simulink model "Multiple"  (R2023a)
settings: Solver=VariableStepAuto  StartTime=0.0  StopTime=1  RelTol=1e-3
settings Model: Creator=Admin  LastModifiedBy=Admin

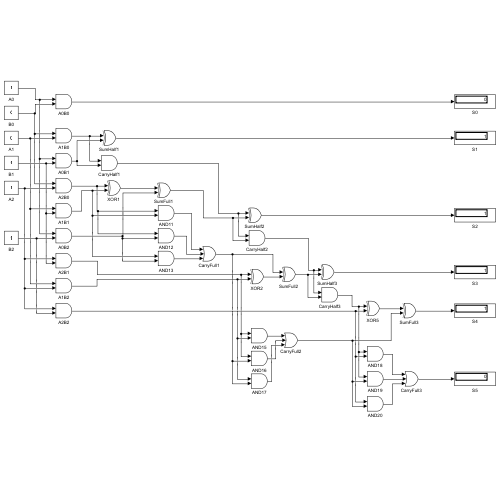
[thumbnail: Simulink's stored preview of the top-level diagram]
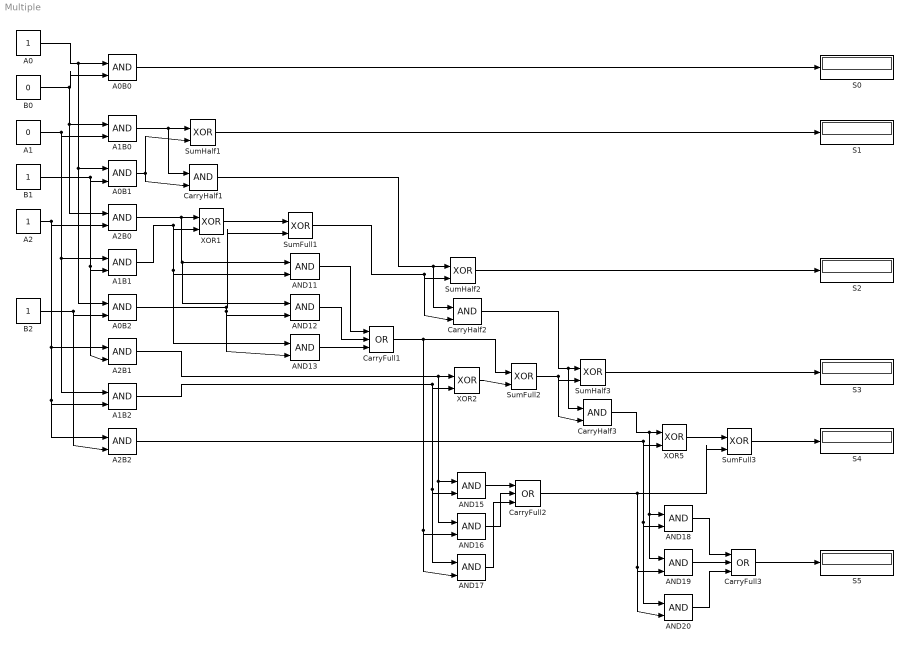
== system Multiple ==
  A0 : Constant  SampleTime=-1
  A0B0 : Logic  IconShape=distinctive  AllPortsSameDT=off  OutDataTypeStr=boolean
  A0B1 : Logic  IconShape=distinctive  AllPortsSameDT=off  OutDataTypeStr=boolean
  A0B2 : Logic  IconShape=distinctive  AllPortsSameDT=off  OutDataTypeStr=boolean
  A1 : Constant  Value=0  SampleTime=-1
  A1B0 : Logic  IconShape=distinctive  AllPortsSameDT=off  OutDataTypeStr=boolean
  A1B1 : Logic  IconShape=distinctive  AllPortsSameDT=off  OutDataTypeStr=boolean
  A1B2 : Logic  IconShape=distinctive  AllPortsSameDT=off  OutDataTypeStr=boolean
  A2 : Constant  SampleTime=-1
  A2B0 : Logic  IconShape=distinctive  AllPortsSameDT=off  OutDataTypeStr=boolean
  A2B1 : Logic  IconShape=distinctive  AllPortsSameDT=off  OutDataTypeStr=boolean
  A2B2 : Logic  IconShape=distinctive  AllPortsSameDT=off  OutDataTypeStr=boolean
  AND{11..13,15..20} (9 alike) : Logic  IconShape=distinctive  AllPortsSameDT=off  OutDataTypeStr=boolean
  B0 : Constant  Value=0  SampleTime=-1
  B1 : Constant  SampleTime=-1
  B2 : Constant  SampleTime=-1
  CarryFull1 : Logic  Operator=OR  Inputs=3  IconShape=distinctive  AllPortsSameDT=off  OutDataTypeStr=boolean
  CarryFull2 : Logic  Operator=OR  Inputs=3  IconShape=distinctive  AllPortsSameDT=off  OutDataTypeStr=boolean
  CarryFull3 : Logic  Operator=OR  Inputs=3  IconShape=distinctive  AllPortsSameDT=off  OutDataTypeStr=boolean
  CarryHalf1 : Logic  IconShape=distinctive  AllPortsSameDT=off  OutDataTypeStr=boolean
  CarryHalf2 : Logic  IconShape=distinctive  AllPortsSameDT=off  OutDataTypeStr=boolean
  CarryHalf3 : Logic  IconShape=distinctive  AllPortsSameDT=off  OutDataTypeStr=boolean
  S{0..5} (6 alike) : Display
  SumFull1 : Logic  Operator=XOR  IconShape=distinctive  AllPortsSameDT=off  OutDataTypeStr=boolean
  SumFull2 : Logic  Operator=XOR  IconShape=distinctive  AllPortsSameDT=off  OutDataTypeStr=boolean
  SumFull3 : Logic  Operator=XOR  IconShape=distinctive  AllPortsSameDT=off  OutDataTypeStr=boolean
  SumHalf1 : Logic  Operator=XOR  IconShape=distinctive  AllPortsSameDT=off  OutDataTypeStr=boolean
  SumHalf2 : Logic  Operator=XOR  IconShape=distinctive  AllPortsSameDT=off  OutDataTypeStr=boolean
  SumHalf3 : Logic  Operator=XOR  IconShape=distinctive  AllPortsSameDT=off  OutDataTypeStr=boolean
  XOR1 : Logic  Operator=XOR  IconShape=distinctive  AllPortsSameDT=off  OutDataTypeStr=boolean
  XOR2 : Logic  Operator=XOR  IconShape=distinctive  AllPortsSameDT=off  OutDataTypeStr=boolean
  XOR5 : Logic  Operator=XOR  IconShape=distinctive  AllPortsSameDT=off  OutDataTypeStr=boolean
  wires:
  A0/1 -> A0B2/1, A0B1/1, A0B0/1
  B0/1 -> A2B0/1, A1B0/1, A0B0/2
  B1/1 -> A2B1/2, A1B1/2, A0B1/2
  A2/1 -> A2B2/1, A1B2/2, A2B1/1, A2B0/2
  A1/1 -> A1B2/1, A1B1/1, A1B0/2
  B2/1 -> A2B2/2, A0B2/2
  A0B0/1 -> S0/1
  A1B0/1 -> CarryHalf1/1, SumHalf1/1
  A0B1/1 -> CarryHalf1/2, SumHalf1/2
  SumHalf1/1 -> S1/1
  A2B0/1 -> AND12/1, AND11/1, XOR1/1
  A1B1/1 -> AND13/1, AND11/2, XOR1/2
  XOR1/1 -> SumFull1/1
  A0B2/1 -> AND13/2, AND12/2, SumFull1/2
  AND12/1 -> CarryFull1/2
  AND11/1 -> CarryFull1/1
  AND13/1 -> CarryFull1/3
  CarryHalf1/1 -> CarryHalf2/1, SumHalf2/1
  SumFull1/1 -> CarryHalf2/2, SumHalf2/2
  SumHalf2/1 -> S2/1
  A2B1/1 -> AND16/1, AND15/1, XOR2/1
  A1B2/1 -> AND17/1, AND15/2, XOR2/2
  XOR2/1 -> SumFull2/2
  CarryFull1/1 -> AND17/2, AND16/2, SumFull2/1
  SumHalf3/1 -> S3/1
  CarryHalf2/1 -> CarryHalf3/1, SumHalf3/1
  SumFull2/1 -> CarryHalf3/2, SumHalf3/2
  AND16/1 -> CarryFull2/2
  AND15/1 -> CarryFull2/1
  AND17/1 -> CarryFull2/3
  A2B2/1 -> AND20/1, AND18/2, XOR5/2
  CarryHalf3/1 -> AND19/1, AND18/1, XOR5/1
  XOR5/1 -> SumFull3/1
  CarryFull2/1 -> AND20/2, AND19/2, SumFull3/2
  SumFull3/1 -> S4/1
  AND19/1 -> CarryFull3/2
  AND18/1 -> CarryFull3/1
  AND20/1 -> CarryFull3/3
  CarryFull3/1 -> S5/1
